simulink model "NMPC_ESNx_ESPLEA"  (R2020b)
settings: Solver=FixedStepDiscrete  StartTime=0.0  StopTime=Time_Stop  FixedStep=Par.Ts  RelTol=1e-3
values from neighbouring files (symbols this model uses):
  dumax = [2  1]'    [CarregaDados.m]
  Hc = 3    [CarregaDados.m]
  head_x0 = 111    [CarregaDados.m]
  Hp = 10    [CarregaDados.m]
  NivelRuido = 2    [CarregaDados.m]
  NivelRuidoHead = 2    [CarregaDados.m]
  NivelRuidoLa = 3    [CarregaDados.m]
  Par = dados_LEA_Par(Ts)    [CarregaDados.m]
  q = [1e2 10]    [CarregaDados.m]
  qm_x0 = 1.87/3600    (= 0.000519444444444)    [CarregaDados.m]
  qu = [0 1]    [CarregaDados.m]
  r = [0.5,1]    [CarregaDados.m]
  Ts = 1    [CarregaDados.m]
  Ts_NMPC = 30    [CarregaDados.m]
  udes = [0 46]'    [CarregaDados.m]
  xmk = [La_x0; pwh_x0; qm_x0; Pin; head_x0; dp_bomba; P_hp_bomba; vazao_choke; qr_res; Par.visc; Par.IP]    [CarregaDados.m]
undefined symbols (not defined in the file or in its folder): Sim_BCS_LEA
libraries: dspsrcs4 x3
settings Model: Creator=odilo  LastModifiedBy=DELL

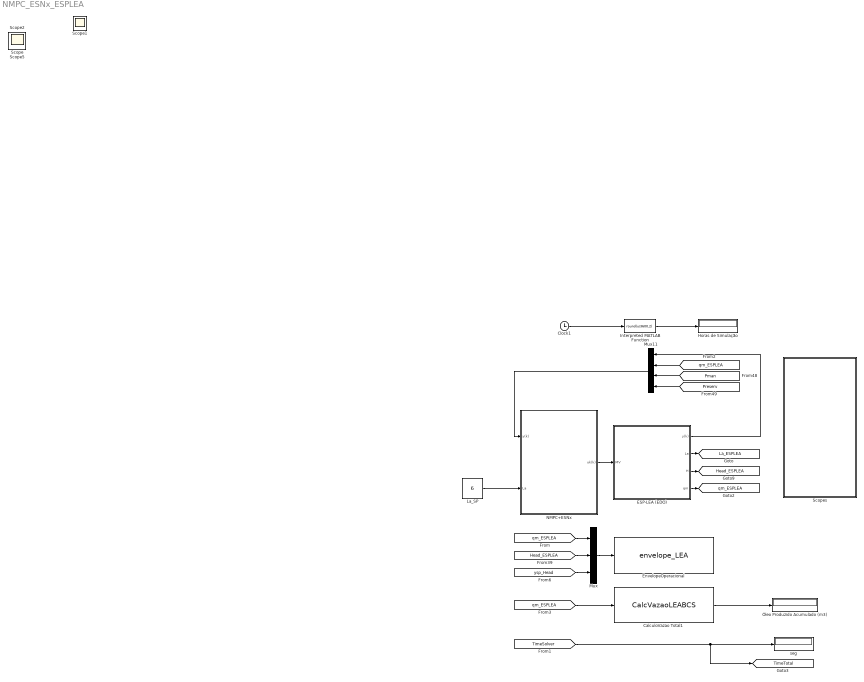
== system NMPC_ESNx_ESPLEA ==
  CalculoVazao Total1 : S-Function  FunctionName=CalcVazaoLEABCS  Parameters=Ts,qm_x0  SFunctionDeploymentMode=off  EnableBusSupport=off
  Clock1 : Clock
  ESP-LEA (EDO) : Subsystem
  EnvelopeOperacional : S-Function  FunctionName=envelope_LEA  Parameters=Par,qm_x0,head_x0  SFunctionDeploymentMode=off  EnableBusSupport=off
  Horas de Simulação : Display
  Interpreted MATLAB Function : MATLABFcn  MATLABFcn=round(u/3600,2)
  La_SP : Constant  Value=6
  Mux : Mux  Inputs=3
  Mux11 : Mux
  NMPC+ESNx : Subsystem
  Scopes : Subsystem
  seg : Display
  Óleo Produzido Acumulado (m3) : Display
  Scope{,1..2,5} (4 alike) : Scope
  tag scope: Head_ESPLEA=global, La_ESPLEA=global, TimeTotal=global, qm_ESPLEA=global
  wires:
  [Pman] -> Mux11/3
  [Preserv] -> Mux11/4
  [qm_ESPLEA] -> Mux11/2
  ESP-LEA (EDO)/1(y(k)) -> Mux11/1
  ESP-LEA (EDO)/3(H) -> [Head_ESPLEA]
  ESP-LEA (EDO)/2(La) -> [La_ESPLEA]
  NMPC+ESNx/1(uk(k)) -> ESP-LEA (EDO)/1(MV)
  ESP-LEA (EDO)/4(qm) -> [qm_ESPLEA]
  Mux11/1 -> NMPC+ESNx/1(y(k))
  [ysp_Head] -> Mux/3
  [TimeSolver] -> [TimeTotal], seg/1
  [qm_ESPLEA] -> Mux/1
  [Head_ESPLEA] -> Mux/2
  Mux/1 -> EnvelopeOperacional/1
  Clock1/1 -> Interpreted MATLAB Function/1
  Interpreted MATLAB Function/1 -> Horas de Simulação/1
  La_SP/1 -> NMPC+ESNx/2(La)
  CalculoVazao Total1/1 -> Óleo Produzido Acumulado (m3)/1
  [qm_ESPLEA] -> CalculoVazao Total1/1

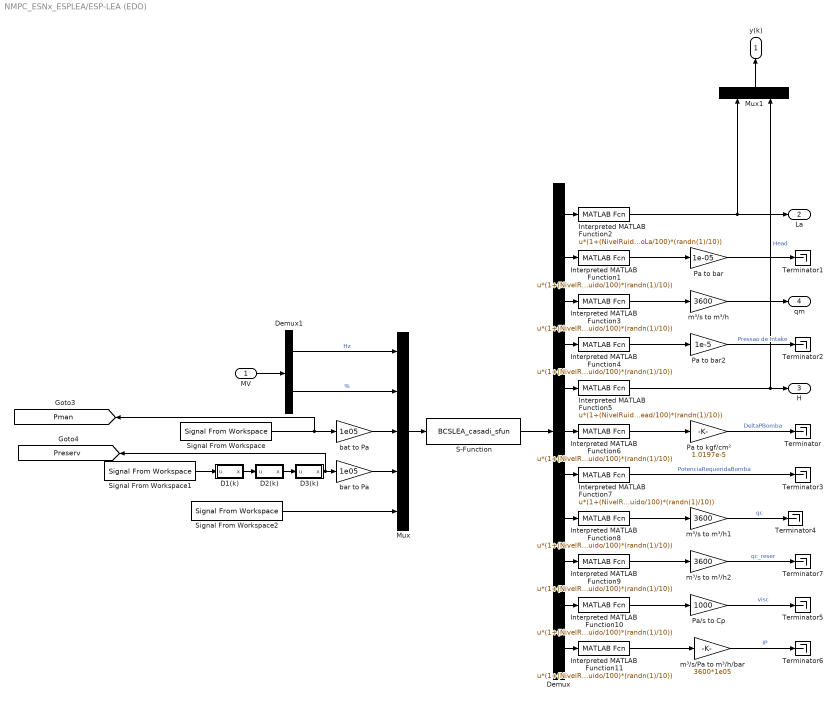
== system NMPC_ESNx_ESPLEA/ESP-LEA (EDO) ==
  MV : Inport
  D1(k) : Subsystem  mask{TIni=20000, DeltaT=60, ValorP=-0.15}
      mask prompts: TIni "Tempo Inicio"; DeltaT "Duracao"; ValorP "Valor da Perturbacao"
  D2(k) : Subsystem  mask{TIni=50000, DeltaT=100, ValorP=0.15}
      mask prompts: TIni "Tempo Inicio"; DeltaT "Duracao"; ValorP "Valor da Perturbacao"
  D3(k) : Subsystem  mask{TIni=90000, DeltaT=60, ValorP=-0.15}
      mask prompts: TIni "Tempo Inicio"; DeltaT "Duracao"; ValorP "Valor da Perturbacao"
  Demux : Demux  Outputs=11
  Demux1 : Demux  Outputs=2
  Interpreted MATLAB Function{1,3..4,6..11} (9 alike) : MATLABFcn  MATLABFcn=u*(1+(NivelRuido/100)*(randn(1)/10))
  Interpreted MATLAB Function2 : MATLABFcn  MATLABFcn=u*(1+(NivelRuidoLa/100)*(randn(1)/10))
  Interpreted MATLAB Function5 : MATLABFcn  MATLABFcn=u*(1+(NivelRuidoHead/100)*(randn(1)/10))
  Mux : Mux  Inputs=5
  Mux1 : Mux  Inputs=2
  Pa to bar : Gain  Gain=1e-05
  Pa to bar2 : Gain  Gain=1e-5
  Pa to kgf/cm² : Gain  Gain=1.0197e-5
  Pa/s to Cp : Gain  Gain=1000
  S-Function : S-Function  FunctionName=BCSLEA_casadi_sfun  Parameters=xmk,Sim_BCS_LEA  SFunctionDeploymentMode=off  EnableBusSupport=off
  Signal From Workspace : dspsrcs4/Signal From Workspace  X=Par.Pman(1:Par.Ts:end)  Ts=Par.Ts  nsamps=1  OutputAfterFinalValue=Setting to zero  ignoreOrWarnInputAndFrameLengths=off  OutputFrames=off
  Signal From Workspace1 : dspsrcs4/Signal From Workspace  X=Par.Resv(1:Par.Ts:end)  Ts=Par.Ts  nsamps=1  OutputAfterFinalValue=Setting to zero  ignoreOrWarnInputAndFrameLengths=off  OutputFrames=off
  Signal From Workspace2 : dspsrcs4/Signal From Workspace  X=Par.Tintake(1:Par.Ts:end)  Ts=Par.Ts  nsamps=1  OutputAfterFinalValue=Setting to zero  ignoreOrWarnInputAndFrameLengths=off  OutputFrames=off
  Terminator{,1..7} (8 alike) : Terminator
  bar to Pa : Gain  Gain=1e05
  bat to Pa : Gain  Gain=1e05
  m³/s to m³/h : Gain  Gain=3600
  m³/s to m³/h1 : Gain  Gain=3600
  m³/s to m³/h2 : Gain  Gain=3600
  "m³/s/Pa to m³/h/bar " : Gain  Gain=3600*1e05
  y(k) : Outport
  La : Outport  Port=2
  H : Outport  Port=3
  qm : Outport  Port=4
  tag scope: Pman=global, Preserv=global
  wires:
  Mux/1 -> S-Function/1
  Demux/2 -> Interpreted MATLAB Function1/1
  Demux/4 -> Interpreted MATLAB Function4/1
  Demux/6 -> Interpreted MATLAB Function6/1
  Demux/7 -> Interpreted MATLAB Function7/1
  Demux/8 -> Interpreted MATLAB Function8/1
  m³/s to m³/h1/1 -> Terminator4/1  "qc"
  Demux/9 -> Interpreted MATLAB Function9/1
  Demux/10 -> Interpreted MATLAB Function10/1
  Demux/11 -> Interpreted MATLAB Function11/1
  Pa to bar2/1 -> Terminator2/1  "Pressao de Intake"
  Pa to kgf/cm²/1 -> Terminator/1  "DeltaPBomba"
  m³/s to m³/h/1 -> qm/1
  Demux/1 -> Interpreted MATLAB Function2/1
  Demux/3 -> Interpreted MATLAB Function3/1
  S-Function/1 -> Demux/1
  Demux/5 -> Interpreted MATLAB Function5/1
  Interpreted MATLAB Function1/1 -> Pa to bar/1
  Interpreted MATLAB Function3/1 -> m³/s to m³/h/1
  Interpreted MATLAB Function4/1 -> Pa to bar2/1
  Interpreted MATLAB Function5/1 -> Mux1/2, H/1  "Head"
  Interpreted MATLAB Function6/1 -> Pa to kgf/cm²/1
  Interpreted MATLAB Function8/1 -> m³/s to m³/h1/1
  Interpreted MATLAB Function9/1 -> m³/s to m³/h2/1
  Interpreted MATLAB Function10/1 -> Pa/s to Cp/1
  Interpreted MATLAB Function11/1 -> "m³/s/Pa to m³/h/bar "/1
  Demux1/2 -> Mux/2  "%"
  bar to Pa/1 -> Mux/4
  bat to Pa/1 -> Mux/3
  MV/1 -> Demux1/1
  Demux1/1 -> Mux/1  "Hz"
  Signal From Workspace/1 -> [Pman], bat to Pa/1
  Interpreted MATLAB Function2/1 -> Mux1/1, La/1
  Signal From Workspace1/1 -> D1(k)/1(u)
  D2(k)/1(x) -> D3(k)/1(u)
  Mux1/1 -> y(k)/1
  D3(k)/1(x) -> bar to Pa/1, [Preserv]
  Signal From Workspace2/1 -> Mux/5
  D1(k)/1(x) -> D2(k)/1(u)
  Pa to bar/1 -> Terminator1/1
  Interpreted MATLAB Function7/1 -> Terminator3/1  "PotenciaRequeridaBomba"
  m³/s to m³/h2/1 -> Terminator7/1  "qc_reser"
  Pa/s to Cp/1 -> Terminator5/1  "visc"
  "m³/s/Pa to m³/h/bar "/1 -> Terminator6/1  "IP"

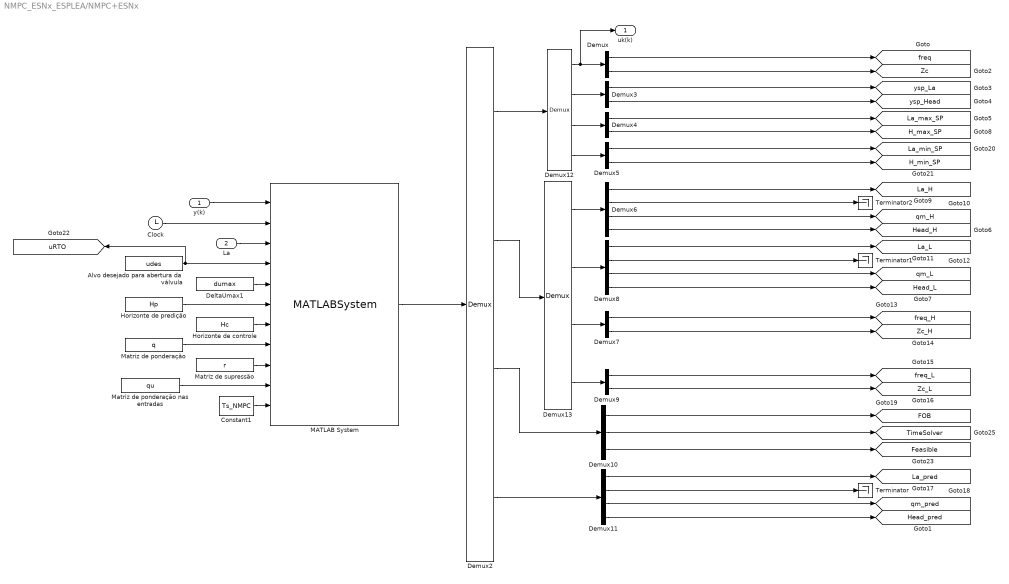
== system NMPC_ESNx_ESPLEA/NMPC+ESNx ==
  y(k) : Inport
  La : Inport  Port=2
  Alvo desejado para abertura da válvula : Constant  Value=udes
  Clock : Clock
  Constant1 : Constant  Value=Ts_NMPC
  DeltaUmax1 : Constant  Value=dumax
  Demux{,3..5,7,9} (6 alike) : Demux  Outputs=2
  Demux10 : Demux  Outputs=3
  Demux11 : Demux
  Demux12 : Demux  Outputs=[2 2 2 2]
  Demux13 : Demux  Outputs=[4 4 2 2]
  Demux2 : Demux  Outputs=[8 12 3 4 ]
  Demux6 : Demux
  Demux8 : Demux
  Horizonte de controle : Constant  Value=Hc
  Horizonte de predição : Constant  Value=Hp
  MATLAB System : MATLABSystem  System=casadi_blockNMPC_ESNx  SimulateUsing=Interpreted execution
      mask Type: casadi_blockNMPC_ESNx
      mask Display:
      | disp('casadi_blockNMPC_ESNx');
      | port_label('input',1,'DadosProcesso');
      | port_label('input',2,'t');
      | port_label('input',3,'SP');
      | port_label('input',4,'uRTO');
      | port_label('input',5,'dumax');
      | port_label('input',6,'Hp');
      | port_label('input',7,'Hc');
      | port_label('input',8,'q');
      | port_label('input',9,'r');
      | port_label('input',10,'qu');
      | port_label('input',11,'PassoMPC');
      | port_label('output',1,'u');
  Matriz de ponderação : Constant  Value=q
  Matriz de ponderação nas entradas : Constant  Value=qu
  Matriz de supressão : Constant  Value=r
  Terminator : Terminator
  Terminator1 : Terminator
  Terminator2 : Terminator
  uk(k) : Outport
  tag scope: FOB=global, Feasible=global, H_max_SP=global, H_min_SP=global, Head_H=global, Head_L=global, Head_pred=global, La_H=global, La_L=global, La_max_SP=global, La_min_SP=global, La_pred=global, TimeSolver=global, Zc=global, Zc_H=global, Zc_L=global, freq=global, freq_H=global, freq_L=global, qm_H=global, qm_L=global, qm_pred=global, uRTO=global, ysp_Head=global, ysp_La=global
  wires:
  Demux6/1 -> [La_H]
  Demux8/2 -> Terminator1/1
  Demux9/2 -> [Zc_L]
  Demux11/3 -> [qm_pred]
  Demux7/2 -> [Zc_H]
  Matriz de ponderação/1 -> MATLAB System/8
  Demux11/2 -> Terminator/1
  Demux6/2 -> Terminator2/1
  Demux4/2 -> [H_max_SP]
  Demux13/2 -> Demux8/1
  Demux2/2 -> Demux13/1
  MATLAB System/1 -> Demux2/1
  Demux13/3 -> Demux7/1
  Demux12/3 -> Demux4/1
  Demux10/2 -> [TimeSolver]
  Demux2/4 -> Demux11/1
  Demux13/4 -> Demux9/1
  Demux12/1 -> uk(k)/1, Demux/1
  Demux13/1 -> Demux6/1
  Demux2/3 -> Demux10/1
  Horizonte de controle/1 -> MATLAB System/7
  Matriz de ponderação nas entradas/1 -> MATLAB System/10
  Demux10/1 -> [FOB]
  Demux/2 -> [Zc]
  Demux2/1 -> Demux12/1
  Demux7/1 -> [freq_H]
  Demux6/3 -> [qm_H]
  Demux12/4 -> Demux5/1
  Demux11/1 -> [La_pred]
  Demux9/1 -> [freq_L]
  Matriz de supressão/1 -> MATLAB System/9
  Demux5/2 -> [H_min_SP]
  Demux10/3 -> [Feasible]
  Demux8/1 -> [La_L]
  Demux8/3 -> [qm_L]
  Demux4/1 -> [La_max_SP]
  Demux11/4 -> [Head_pred]
  Demux5/1 -> [La_min_SP]
  Demux8/4 -> [Head_L]
  Demux6/4 -> [Head_H]
  Demux3/1 -> [ysp_La]
  Demux3/2 -> [ysp_Head]
  Demux12/2 -> Demux3/1
  Demux/1 -> [freq]
  Clock/1 -> MATLAB System/2
  Constant1/1 -> MATLAB System/11
  Horizonte de predição/1 -> MATLAB System/6
  y(k)/1 -> MATLAB System/1
  La/1 -> MATLAB System/3
  Alvo desejado para abertura da válvula/1 -> [uRTO], MATLAB System/4
  DeltaUmax1/1 -> MATLAB System/5

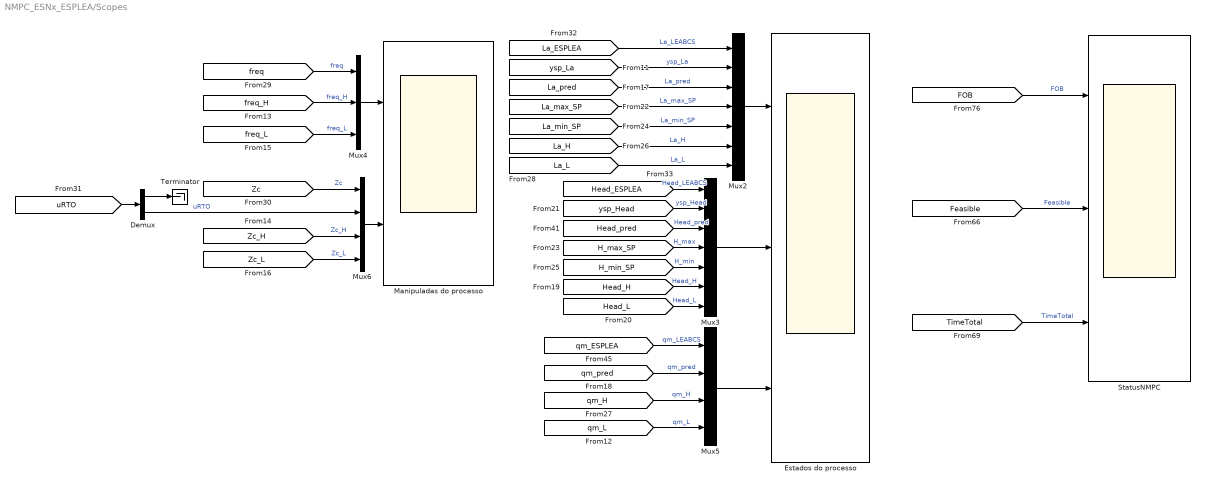
== system NMPC_ESNx_ESPLEA/Scopes ==
  Demux : Demux  Outputs=2
  Estados do processo : Scope  NumInputPorts=3
  Manipuladas do processo : Scope  NumInputPorts=2
  Mux2 : Mux  Inputs=7
  Mux3 : Mux  Inputs=7
  Mux4 : Mux  Inputs=3
  Mux5 : Mux
  Mux6 : Mux
  StatusNMPC : Scope  NumInputPorts=3
  Terminator : Terminator
  wires:
  [TimeTotal] -> StatusNMPC/3  "TimeTotal"
  [Zc_H] -> Mux6/3  "Zc_H"
  Mux4/1 -> Manipuladas do processo/1
  Mux6/1 -> Manipuladas do processo/2
  [Zc_L] -> Mux6/4  "Zc_L"
  Mux3/1 -> Estados do processo/2
  [freq_L] -> Mux4/3  "freq_L"
  Mux5/1 -> Estados do processo/3
  [freq_H] -> Mux4/2  "freq_H"
  Mux2/1 -> Estados do processo/1
  [Zc] -> Mux6/1  "Zc"
  [FOB] -> StatusNMPC/1  "FOB"
  [freq] -> Mux4/1  "freq"
  [Feasible] -> StatusNMPC/2  "Feasible"
  [uRTO] -> Demux/1
  Demux/2 -> Mux6/2  "uRTO"
  Demux/1 -> Terminator/1
  [La_ESPLEA] -> Mux2/1  "La_LEABCS"
  [ysp_La] -> Mux2/2  "ysp_La"
  [La_pred] -> Mux2/3  "La_pred"
  [La_max_SP] -> Mux2/4  "La_max_SP"
  [La_min_SP] -> Mux2/5  "La_min_SP"
  [La_H] -> Mux2/6  "La_H"
  [La_L] -> Mux2/7  "La_L"
  [Head_ESPLEA] -> Mux3/1  "Head_LEABCS"
  [ysp_Head] -> Mux3/2  "ysp_Head"
  [Head_pred] -> Mux3/3  "Head_pred"
  [H_max_SP] -> Mux3/4  "H_max"
  [Head_L] -> Mux3/7  "Head_L"
  [Head_H] -> Mux3/6  "Head_H"
  [H_min_SP] -> Mux3/5  "H_min"
  [qm_L] -> Mux5/4  "qm_L"
  [qm_H] -> Mux5/3  "qm_H"
  [qm_pred] -> Mux5/2  "qm_pred"
  [qm_ESPLEA] -> Mux5/1  "qm_LEABCS"

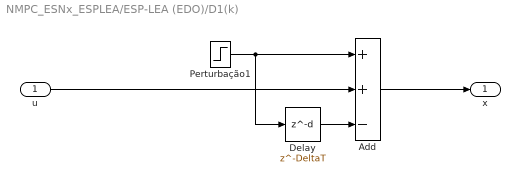
== system NMPC_ESNx_ESPLEA/ESP-LEA (EDO)/D1(k) ==
  u : Inport
  Add : Sum  Inputs=++-
  Delay : Delay  DelayLength=DeltaT
  Perturbação1 : Step  Time=TIni  After=ValorP  SampleTime=0
  x : Outport
  wires:
  Perturbação1/1 -> Delay/1, Add/1
  Add/1 -> x/1
  Delay/1 -> Add/3
  u/1 -> Add/2

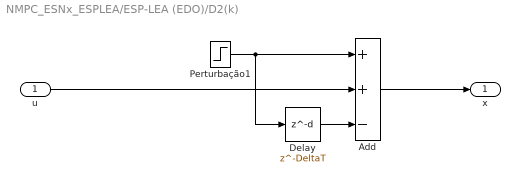
== system NMPC_ESNx_ESPLEA/ESP-LEA (EDO)/D2(k) ==
  u : Inport
  Add : Sum  Inputs=++-
  Delay : Delay  DelayLength=DeltaT
  Perturbação1 : Step  Time=TIni  After=ValorP  SampleTime=0
  x : Outport
  wires:
  Perturbação1/1 -> Delay/1, Add/1
  Add/1 -> x/1
  Delay/1 -> Add/3
  u/1 -> Add/2

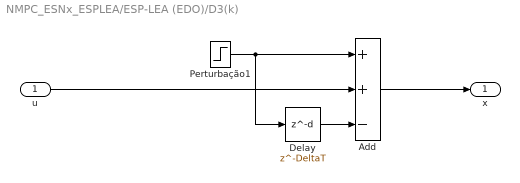
== system NMPC_ESNx_ESPLEA/ESP-LEA (EDO)/D3(k) ==
  u : Inport
  Add : Sum  Inputs=++-
  Delay : Delay  DelayLength=DeltaT
  Perturbação1 : Step  Time=TIni  After=ValorP  SampleTime=0
  x : Outport
  wires:
  Perturbação1/1 -> Delay/1, Add/1
  Add/1 -> x/1
  Delay/1 -> Add/3
  u/1 -> Add/2
